simulink model "rigspace"  (Simulink 5.0)
settings: Solver=ode45  StartTime=0.0  StopTime=300.0  RelTol=1e-3
libraries: simulink x1

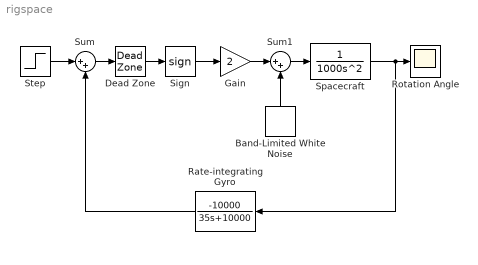
== system rigspace ==
  Band-Limited White Noise : simulink/Sources/Band-Limited White Noise  Orientation=up  Cov=[0.01]  Ts=0.01  seed=[1000]
  Dead Zone : DeadZone  LowerValue=-0.2  UpperValue=0.2  SaturateOnIntegerOverflow=on
  Gain : Gain  Gain=2  SaturateOnIntegerOverflow=on
  Rate-integrating Gyro : TransferFcn  Orientation=left  Numerator=-10000  Denominator=[35 10000]
  Rotation Angle : Scope
      settings: SaveName=theta2  DataFormat=Array  MaxDataPoints=15000
  Sign : Signum
  Spacecraft : TransferFcn  Denominator=[1000 0 0]
  Step : Step  Time=0  After=0.1  SampleTime=0
  Sum : Sum  Inputs=|++  SaturateOnIntegerOverflow=on
  Sum1 : Sum  Inputs=|++  SaturateOnIntegerOverflow=on
  wires:
  Sum1/1 -> Spacecraft/1
  Band-Limited White Noise/1 -> Sum1/2
  Spacecraft/1 -> Rotation Angle/1, Rate-integrating Gyro/1
  Step/1 -> Sum/1
  Gain/1 -> Sum1/1
  Sum/1 -> Dead Zone/1
  Dead Zone/1 -> Sign/1
  Sign/1 -> Gain/1
  Rate-integrating Gyro/1 -> Sum/2
